simulink model "ExampleVariantSubsystem"  (R2017b)
settings: Solver=VariableStepAuto  StartTime=0.0  StopTime=10.0  RelTol=1e-3
settings Model: Creator=aarrieta  LastModifiedBy=aarrieta

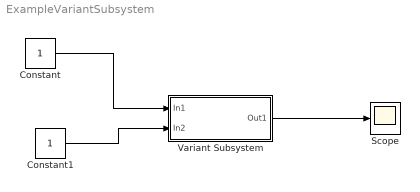
== system ExampleVariantSubsystem ==
  Constant : Constant
  Constant1 : Constant
  Scope : Scope
  Variant Subsystem : Subsystem  Variant=on
  wires:
  Constant/1 -> Variant Subsystem/1(In1)
  Constant1/1 -> Variant Subsystem/2(In2)
  Variant Subsystem/1(Out1) -> Scope/1

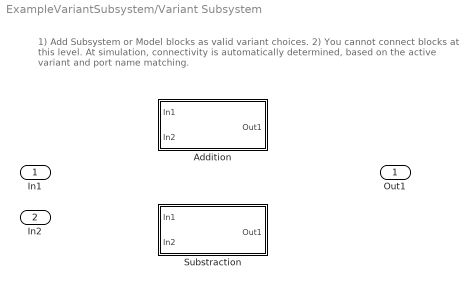
== system ExampleVariantSubsystem/Variant Subsystem ==
  note: 1) Add Subsystem or Model blocks as valid variant choices.
      | 2) You cannot connect blocks at this level. At simulation, connectivity is automatically
      | determined, based on the active variant and port name matching.
  In1 : Inport
  In2 : Inport  Port=2
  Addition : Subsystem  VariantControl=Addition
  Substraction : Subsystem  VariantControl=Substraction
  Out1 : Outport

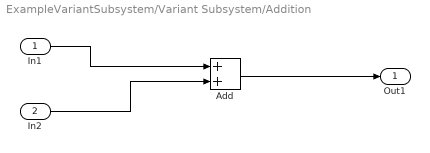
== system ExampleVariantSubsystem/Variant Subsystem/Addition ==
  In1 : Inport
  In2 : Inport  Port=2
  Add : Sum
  Out1 : Outport
  wires:
  In2/1 -> Add/2
  In1/1 -> Add/1
  Add/1 -> Out1/1

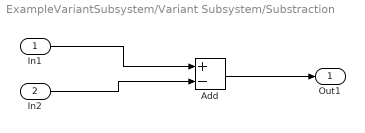
== system ExampleVariantSubsystem/Variant Subsystem/Substraction ==
  In1 : Inport
  In2 : Inport  Port=2
  Add : Sum  Inputs=+-
  Out1 : Outport
  wires:
  In1/1 -> Add/1
  In2/1 -> Add/2
  Add/1 -> Out1/1
